simulink model "dspfsinecomp"  (Simulink 4.00)
settings: Solver=FixedStepDiscrete  StartTime=0.0  StopTime=inf  RelTol=1e-3
libraries: dspstat3 x4, dspsrcs3 x3
Description:
  | Comparison of frame-based sine wave generation techniques.
settings Model: Creator=don  LastModifiedBy=asharma  SaveTime=off  SaveOutput=off  LimitDataPoints=off  IntegerOverflowMsg=none  RTWOptions=-aRollThreshold=2  ExtModeTrigMode=oneshot  ExtModeArmWhenConnect=off  BlockReductionOpt=off

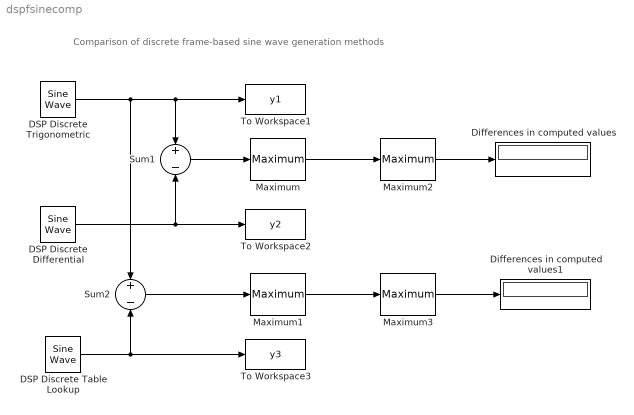
== system dspfsinecomp ==
  note: Comparison of discrete frame-based
      | sine wave generation methods
  DSP Discrete Differential : dspsrcs3/Sine Wave  Amplitude=1  Frequency=1e4  Phase=0  SampleMode=Discrete  OutComplex=Real  CompMethod=Differential  SampleTime=1e-5  SamplesPerFrame=32  ResetState=Restart at time zero
  DSP Discrete Table Lookup : dspsrcs3/Sine Wave  Amplitude=1  Frequency=1e4  Phase=0  SampleMode=Discrete  OutComplex=Real  CompMethod=Table Lookup  SampleTime=1e-5  SamplesPerFrame=32  ResetState=Restart at time zero
  DSP Discrete Trigonometric : dspsrcs3/Sine Wave  Amplitude=1  Frequency=1e4  Phase=0  SampleMode=Discrete  OutComplex=Real  CompMethod=Trigonometric Fcn  SampleTime=1e-5  SamplesPerFrame=32  ResetState=Restart at time zero
  Differences in computed values : Display
      settings: Format=short
  Differences in computed values1 : Display
      settings: Format=short
  Maximum : dspstat3/Maximum  fcn=Running  reset=None
  Maximum1 : dspstat3/Maximum  fcn=Running  reset=None
  Maximum2 : dspstat3/Maximum  fcn=Value  reset=None
  Maximum3 : dspstat3/Maximum  fcn=Value  reset=None
  Sum1 : Sum  Inputs=+-  SaturateOnIntegerOverflow=on
  Sum2 : Sum  Inputs=+-  SaturateOnIntegerOverflow=on
  To Workspace1 : ToWorkspace  VariableName=y1  SampleTime=-1  SaveFormat=Array
  To Workspace2 : ToWorkspace  VariableName=y2  SampleTime=-1  SaveFormat=Array
  To Workspace3 : ToWorkspace  VariableName=y3  SampleTime=-1  SaveFormat=Array
  wires:
  DSP Discrete Trigonometric/1 -> Sum1/1, To Workspace1/1, Sum2/1
  Sum1/1 -> Maximum/1
  Maximum/1 -> Maximum2/1
  DSP Discrete Differential/1 -> Sum1/2, To Workspace2/1
  Sum2/1 -> Maximum1/1
  DSP Discrete Table Lookup/1 -> Sum2/2, To Workspace3/1
  Maximum1/1 -> Maximum3/1
  Maximum2/1 -> Differences in computed values/1
  Maximum3/1 -> Differences in computed values1/1
